simulink model "simmm"  (R2020b)
settings: Solver=ode15s  StartTime=0.0  StopTime=20  FixedStep=1e-3
libraries: simulink x1
settings Model: Creator=mehme  LastModifiedBy=mehme

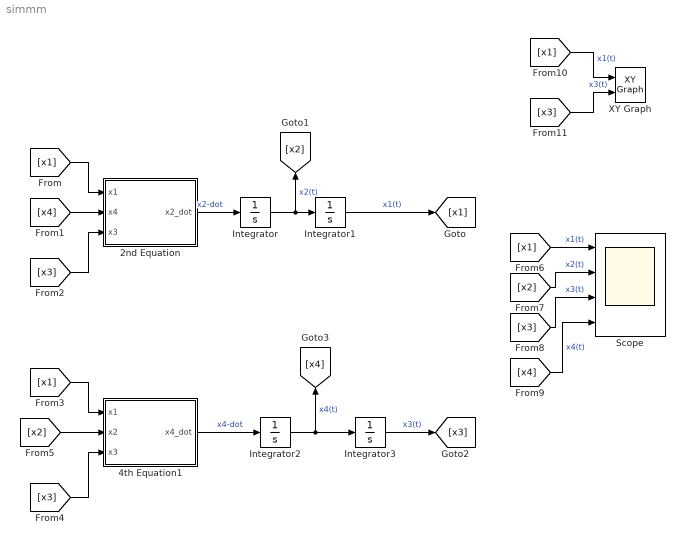
== system simmm ==
  2nd Equation : MATLAB Function  TreatAsAtomicUnit=on
  4th Equation1 : MATLAB Function  TreatAsAtomicUnit=on
  Integrator : Integrator
  Integrator1 : Integrator  InitialCondition=1.2
  Integrator2 : Integrator  InitialCondition=-1.0494
  Integrator3 : Integrator
  Scope : Scope  NumInputPorts=4
  XY Graph : simulink/Sinks/XY Graph  xmin=-2  xmax=1.5  ymin=-1  ymax=1  st=-1
  wires:
  [x1] -> 2nd Equation/1(x1)
  [x4] -> 2nd Equation/2(x4)
  [x3] -> 2nd Equation/3(x3)
  2nd Equation/1(x2_dot) -> Integrator/1  "x2-dot"
  Integrator/1 -> [x2], Integrator1/1  "x2(t)"
  Integrator1/1 -> [x1]  "x1(t)"
  [x2] -> 4th Equation1/2(x2)
  [x1] -> 4th Equation1/1(x1)
  [x3] -> 4th Equation1/3(x3)
  Integrator2/1 -> Integrator3/1, [x4]  "x4(t)"
  4th Equation1/1(x4_dot) -> Integrator2/1  "x4-dot"
  Integrator3/1 -> [x3]  "x3(t)"
  [x1] -> Scope/1  "x1(t)"
  [x2] -> Scope/2  "x2(t)"
  [x3] -> Scope/3  "x3(t)"
  [x4] -> Scope/4  "x4(t)"
  [x1] -> XY Graph/1  "x1(t)"
  [x3] -> XY Graph/2  "x3(t)"

== matlab function simmm/2nd Equation ==
  data: x1 input; x2_dot output; x4 input; x3 input
function x2_dot = fcn(x1,x4,x3)
nu=1/82.45;
nustar=1-nu;

denum1=(sqrt((x1+nu)^2+x3^2))^3;
denum2=(sqrt((x1-nustar)^2+x3^2))^3;
x2_dot = 2*x4+x1-nustar*(x1+nu)/denum1-nu*(x1-nustar)/denum2 ;

== matlab function simmm/4th Equation1 ==
  data: x1 input; x4_dot output; x2 input; x3 input
function x4_dot = fcn(x1,x2,x3)
nu=1/82.45;
nustar=1-nu;

denum1=(sqrt((x1+nu)^2+x3^2))^3;
denum2=(sqrt((x1-nustar)^2+x3^2))^3;
x4_dot = -2*x2+x3-nustar*(x3/denum1)-nu*(x3/denum2) ;
